simulink model "ScanMatcher_v21"  (R2021a)
settings: Solver=FixedStepAuto  StartTime=0.0  StopTime=inf  RelTol=1e-3
model workspace (MAT data in the model file):
  SL_ROS_VariableLengthArrays_MaxSizes : object (value not decoded)
undefined symbols (not defined in the file): Header, Pose, Theta, X, Y
libraries: robotlib x23, robotcorelib x2
(part 2 of 2)

== matlab function ScanMatcher_v21/Precise Localization/Compute Transformation/TrdICP_PP_corr/MATLAB Function4 ==
  data: data_set input size=[2,2000]; model_set input size=[2,2000]; N_d input size=1 [..2000]; N_m input size=1 [..2000]; iterCount output; R output; B_init input; maxIter input; T output; dev_A output; sigmaMult input; alphaIn input; scanTime input; ScanTime output
function [iterCount,R,T,dev_A,ScanTime] = FindTransform(data_set,model_set,N_d,N_m,B_init,maxIter,sigmaMult,alphaIn,scanTime)
%%%%%%%%%%%%%%%%%%%%%%%%%%%%%%%%%%%%%%%%%%%%%%%%%%%%%%%%%%%%%%%%%%%%%%%%%%%
%%%%%%%%%%%%%%%% Rigid ICP, Correntropy, Point to Point %%%%%%%%%%%%%%%%%%%
%%%%%%%%%%%%%%%%%%%%%%%%%%%%%%%%%%%%%%%%%%%%%%%%%%%%%%%%%%%%%%%%%%%%%%%%%%%
% Author  : Abdurrahman YILMAZ
% Date    : 15.09.2021
% Version : v01
% Notes   : ICP based 2D pose estimator. It takes model and data 
% clouds in 2D, target pose and initial pose information, and estimates 
% current pose
%%%%%%%%%%%%%%%%%%%%%%%%%%%%%%%%%%%%%%%%%%%%%%%%%%%%%%%%%%%%%%%%%%%%%%%%%%
    
    if isempty(maxIter) || isnan(maxIter) || isinf(maxIter) || maxIter <= 0 || maxIter >= 500
        maxNumIter = int32(100); % default value
    else
        maxNumIter = maxIter; % taken as ros paramter
    end
    
    if isempty(sigmaMult) || isnan(sigmaMult) || isinf(sigmaMult) || sigmaMult <= 0 || sigmaMult >= 100
        sigmaMultiplier = double(1); % default value
    else
        sigmaMultiplier = sigmaMult; % taken as ros paramter
    end
    
    if isempty(alphaIn) || isnan(alphaIn) || isinf(alphaIn) || alphaIn <= 0 || alphaIn >= 1
        alpha = double(0.8); % default value
    else
        alpha = alphaIn; % taken as ros paramter
    end
    
    sigma = 1;
    sigma_km1 = 0.1;
    B_km1 = B_init;
    B_k = B_init;
    count_stop_iter = 0;
    iterCount = int16(0);
    
    model_in = model_set';
    data_in = data_set';
    
%     N_model = nnz(~isnan(model_in))/2;
%     N_data = nnz(~isnan(data_in))/2;
    
    N_model = N_m;
    N_data = N_d;
    model= model_in(1:N_model,:);
    M1 = model;
    M = [M1,ones(size(M1,1),1)];
    data = data_in(1:N_data,:);
    P1 = data;
    P = [P1,ones(size(P1,1),1)];
    g = zeros(1,size(P1,1));
    
    p_k = zeros(size(P1,1),1);
    Q = zeros(size(P1,1),2);
    X = zeros(size(P1,1),2);
        
%     p_k = zeros(N_data,1);
    mck = [];
    P_trim = [];
    
    for iter = 1:maxNumIter
        iterCount = iterCount + 1;
        Pbar = (B_km1*P')';
        [Idx,Dist] = knnsearch(M(:,1:2),Pbar(:,1:2),'k',1);
        corr_points = [double(Idx),Dist,Pbar,P];
        corr_points = sortrows(corr_points,2);
        
        filterOutDist = median(Dist) + (median(Dist)-min(Dist));
        
        indexId = size(corr_points,1);
        
        for j = size(corr_points,1):-1:1
            if corr_points(j,2) <= filterOutDist
                indexId = j;
                break;
            end
        end
        Idx_filtered = corr_points(1:indexId,1);
        
        mck = [zeros(size(Idx_filtered,1),2),ones(size(Idx_filtered,1),1)];
        mck(:,1:2) = M(Idx_filtered,1:2);
        Pbar_trim = corr_points(1:indexId,3:4);
        P_trim = corr_points(1:indexId,6:8);
        
        DiffModelData = zeros(length(Pbar_trim),1);
        for i=1:1:length(Pbar_trim)
            DiffModelData(i,1)=sqrt((Pbar_trim(i,1)-mck(i,1))^2+(Pbar_trim(i,2)-mck(i,2))^2);
        end
%         if  iter < 100
%             sigma = sigmaMultiplier*std(DiffModelData);
%         else
%             sigma = sigma_km1*alpha + sigmaMultiplier*(1 - alpha)*sqrt(3/kurtosis(DiffModelData)*std(DiffModelData)^2); % 3 is standard Gaussian curve kurtosis 
%         end
        
        if iter ==1
            sigma = sigmaMultiplier*median(DiffModelData)*alpha + (1 - alpha)*sqrt(3/kurtosis(DiffModelData)*std(DiffModelData)^2);
        else
            sigma = sigma_km1*alpha;
        end
        
        for j = 1:1:size(P_trim,1)
            p_k(j) = exp(-(norm(B_km1*P_trim(j,:)'-mck(j,:)')^2/(2*sigma^2)));
        end
        
        sum_p_k_x = zeros(1,2);
        sum_p_k = 0;
        sum_p_k_y = zeros(1,2);
        
        for t = 1:1:size(P_trim,1)
            sum_p_k_x = sum_p_k_x + p_k(t)*P_trim(t,1:2);
            sum_p_k = sum_p_k + p_k(t);
            sum_p_k_y = sum_p_k_y + p_k(t)*mck(t,1:2);
        end
        
        Q_rem = sum_p_k_x/sum_p_k;
        X_rem = sum_p_k_y/sum_p_k;
        
        for tt = 1:1:size(P_trim,1)
            Q(tt,:) = P_trim(tt,1:2) - Q_rem;
            X(tt,:) = mck(tt,1:2) - X_rem;
        end
        
        for i = 1:1:size(P_trim,1)
            g(i) = exp(-(norm(B_km1*[Q(i,:)';1]-[X(i,:)';1])^2/(2*sigma^2)));
        end
        
        D_g = diag(g);
        Ltr_R = -(X'*D_g*Q)/(sigma^2);
        [U,~,Vtr] = svd(Ltr_R);
        if det(X'*D_g*Q) > 0
            D_d_inv = -eye(2);
        else
            D_d_inv = [1,0;0,-1];
        end
        R_k = U*D_d_inv*Vtr;
%         R_k = U*Vtr;
        
        if det(R_k) < 0
            Vtr(:,end) = -Vtr(:,end); 
            R_k = U*D_d_inv*Vtr;
        end
        
        sumForTk = zeros(2,1);
        for p = 1:1:size(P_trim,1)
            sumForTk = sumForTk + (mck(p,1:2)'-R_k*P_trim(p,1:2)')*p_k(p);
        end
        
        t_k = sumForTk/sum_p_k;
        B_k = [R_k,t_k;0,0,1];
%         B_k = [R_k*B_km1(1:2,1:2),R_k*B_km1(1:2,3)+t_k;zeros(1,2),ones(1,1)];
                
        if abs(norm(B_km1(1:3,1:3))-norm(B_k(1:3,1:3))) < 0.00005
            count_stop_iter = count_stop_iter + 1;
            if count_stop_iter > 5
                break;
            end
        else
            count_stop_iter = 0;
        end
        
        B_km1 = B_k(1:3,1:3);
        sigma_km1 = sigma;
    end
        
    B_final = B_k(1:3,1:3);
    
    % Rigid transformation R matrix and T vector
    R = B_final(1:2,1:2);
    T = B_final(1:2,3);
    dev_A = 0;
    iterCount = int16(iterCount);
    ScanTime = scanTime;

== matlab function ScanMatcher_v21/Precise Localization/OdomArray/MATLAB Function3 ==
  data: ScanEstimTime input; OdomArray input; xyth_odom output
function xyth_odom  = OdomUpdater(ScanEstimTime,OdomArray)

    scanTime = ScanEstimTime(1,1);
    
    estimTime = ScanEstimTime(2,1);
    
    indexOdomLast = 1;
    indexOdomFirst = 1;
    th = 0;
    x = 0;
    y = 0;
    
    for i = 1:1:size(OdomArray,1)
        if estimTime >= OdomArray(i,1)
            indexOdomLast = i;
            break;
        end
    end
    
    for i = 1:1:size(OdomArray,1)
        if scanTime >= OdomArray(i,1)
             indexOdomFirst = i;
             break;
        end
    end
    
    if indexOdomLast < indexOdomFirst
        for j = 0:1:indexOdomFirst-indexOdomLast
            if j == 0
                delta_t = OdomArray(indexOdomFirst - 1,1) - scanTime;
            elseif j == indexOdomFirst-indexOdomLast
                delta_t = estimTime - OdomArray(indexOdomLast,1);    
            else
                delta_t = OdomArray(indexOdomFirst - j - 1,1) - OdomArray(indexOdomFirst - j,1);
            end
            v_x = OdomArray(indexOdomFirst - j,2);
            w_z = OdomArray(indexOdomFirst - j,3);
            delta_x = v_x*cos(th)*delta_t;
            delta_y = v_x*sin(th)*delta_t;
            delta_th = w_z*delta_t;
            x = x + delta_x;
            y = y + delta_y;
            th = th + delta_th;
        end
    elseif indexOdomLast == indexOdomFirst
        delta_t = estimTime - scanTime;
        v_x = OdomArray(indexOdomFirst,2);
        w_z = OdomArray(indexOdomFirst,3);
        delta_x = v_x*cos(th)*delta_t;
        delta_y = v_x*sin(th)*delta_t;
        delta_th = w_z*delta_t;
        x = x + delta_x;
        y = y + delta_y;
        th = th + delta_th;
    end
   
%     odomDiff = odomLast - odomInit;
%     x_up = x + odomDiff(1,1);
%     y_up = y + odomDiff(1,1);
%     th_up = wrapTo360(th + odomDiff(1,1));
    
    xyth_odom = [x,y,th];
    
end

== matlab function ScanMatcher_v21/Precise Localization/Publish pose_estim_now_odom_updated (x,y,theta)/MATLAB Function3 ==
  data: x input; y input; x_up output; th input; xyth_odom input; y_up output; th_up output; R_th_up output
function [x_up,y_up,th_up,R_th_up]  = OdomUpdater(x,y,th,xyth_odom)

    xy_up = [cosd(th) -sind(th);sind(th) cosd(th)]*xyth_odom(1,1:2)' + [x;y];
    th_up = wrapTo360(th + rad2deg(xyth_odom(1,3)));
    x_up = xy_up(1,1);
    y_up = xy_up(2,1);
    R_th_up = rotz(th_up);
    
end

== matlab function ScanMatcher_v21/Precise Localization/Extract Model and Data Sets/MATLAB Function1 ==
  data: Sec input; sec output size=1 [..2000]; nSec input
function sec = TimeCalc(Sec,nSec)

    sec = Sec + 10^(-9)*nSec;
end

== matlab function ScanMatcher_v21/Precise Localization/Publish pose_estim_now_with_stamp (x,y,theta,time,frameID,...)/MATLAB Function1 ==
  data: ScanTime input; scanTime output; Sec input; estimTime output size=1 [..2000]; nSec input
function [scanTime,estimTime] = ScanvsEstimTime(ScanTime,Sec,nSec)

    estimTime = Sec + 10^(-9)*nSec;
    scanTime = ScanTime;
end

== matlab function ScanMatcher_v21/Precise Localization/Publish pose_estim_now_with_stamp (x,y,theta,time,frameID,...)/MATLAB Function2 ==
  data: dev_A input; covarianceMatrix output
function covarianceMatrix  = CovarianceEstim(dev_A)
    var_A = dev_A^2;
    x_cov = var_A;
    y_cov = var_A;
    z_cov = 0;
    rotx_cov = 0;
    roty_cov = 0;
    rotz_cov = var_A;

    covarianceMatrix = double([x_cov,0,0,0,0,0 ...
        0,y_cov,0,0,0,0,...
        0,0,z_cov,0,0,0,...
        0,0,0,rotx_cov,0,0,...
        0,0,0,0,roty_cov,0,...
        0,0,0,0,0,rotz_cov]);
end

== matlab function ScanMatcher_v21/Precise Localization/Publish pose_estim_now_odom_updated_with_stamp (x,y,theta,time,frameID,...)/MATLAB Function4 ==
  data: Rin input; x output; y output; z output; w output
function [x,y,z,w]  = Quat(Rin)
    w = Rin(1,1);
    x = Rin(2,1);
    y = Rin(3,1);
    z = Rin(4,1);
end

== matlab function ScanMatcher_v21/Precise Localization/Publish pose_estim_now_odom_updated_with_stamp (x,y,theta,time,frameID,...)/MATLAB Function2 ==
  data: dev_A input; covarianceMatrix output
function covarianceMatrix  = CovarianceEstim(dev_A)
    var_A = dev_A^2;
    x_cov = var_A;
    y_cov = var_A;
    z_cov = 0;
    rotx_cov = 0;
    roty_cov = 0;
    rotz_cov = var_A;

    covarianceMatrix = double([x_cov,0,0,0,0,0 ...
        0,y_cov,0,0,0,0,...
        0,0,z_cov,0,0,0,...
        0,0,0,rotx_cov,0,0,...
        0,0,0,0,roty_cov,0,...
        0,0,0,0,0,rotz_cov]);
end

== matlab function ScanMatcher_v21/Precise Localization/OdomArray/MATLAB Function5 ==
  data: pos_x input; pos_y input; pos_th input; Sec input; nSec input; vel_x input; vel_w_z input; ArrayOdomLast input; ArrayOdomNow output
function ArrayOdomNow  = OdomDataList(pos_x,pos_y,pos_th,Sec,nSec,vel_x,vel_w_z,ArrayOdomLast)

    sec = Sec + 10^(-9)*nSec;
    v_x = vel_x;
    w_z = vel_w_z;
    
    ArrayOdomDummy = ArrayOdomLast;
    
    if sec ~= ArrayOdomLast(1,1)
        ArrayOdomDummy = [sec,v_x,w_z,pos_x,pos_y,pos_th;ArrayOdomDummy(1:end-1,:)];
    end
    
    ArrayOdomNow = ArrayOdomDummy;
    
end

== matlab function ScanMatcher_v21/MATLAB Function8 ==
  data: docking_enable_msg input; docking_state output
function docking_state = Docking_State(docking_enable_msg)
    
    if isempty(docking_enable_msg) || isnan(docking_enable_msg)
        docking_state = false(1);
    else
        if docking_enable_msg
            docking_state = true(1);
        else
            docking_state = false(1);
        end
    end
end

== matlab function ScanMatcher_v21/Precise Localization/Target Pose - Initial Transform/MATLAB Function1 ==
  data: pose_target input; B_init output [..2000]; pose_estim_pre input
function B_init = Initial_tf(pose_target,pose_estim_pre)

    th_B = wrapTo360(pose_estim_pre(3,1)-pose_target(3,1));
%     R_B = [cosd(th_B),-sind(th_B);sind(th_B),cosd(th_B)];
    R_trgt2ref_cf = [cosd(pose_target(3,1)),-sind(pose_target(3,1));sind(pose_target(3,1)),cosd(pose_target(3,1))];
    t_B = R_trgt2ref_cf'*(pose_estim_pre(1:2,1) - pose_target(1:2,1));
%     B_init = [R_B,t_B;0,0,1];
    B_init = rotz(th_B);
    B_init(1:2,3) = t_B;

end

== matlab function ScanMatcher_v21/Precise Localization/Extract Model and Data Sets/MATLAB Function ==
  data: NumberOfPointsInScan input size=1 [..2000]; rangeMax input; rangeMin input; Ranges_data input; Ranges_model input; RangesXY_data output double size=[2,2000]; angle_min input; angle_inc input; RangesXY_model output size=[2,2000]; N_data output size=1 [..2000]; N_model output size=1 [..2000]
function [RangesXY_data,RangesXY_model,N_data,N_model] = Model_Data_Extract(NumberOfPointsInScan,rangeMax,rangeMin,Ranges_data,Ranges_model,angle_min,angle_inc)
    
    N_model = 0;
    N_data = 0;

    if ~isnan(NumberOfPointsInScan)
        Ranges_data(Ranges_data < rangeMin | Ranges_data > rangeMax) = NaN;
        Ranges_model(Ranges_model < rangeMin | Ranges_model > rangeMax) = NaN;
        Ranges_Used_data = double(Ranges_data');            
        RangesXY_data = NaN(2,size(Ranges_Used_data,2));
        Ranges_Used_model = double(Ranges_model');          
        RangesXY_model = NaN(2,size(Ranges_Used_model,2));
%         coder.varsize('RangesXY',[2,2000],[1,1])        
    
        for i = 1:1:NumberOfPointsInScan
            if isinf(Ranges_Used_data(1,i))
               Ranges_Used_data(1,i) = NaN;  
            end
            RangesXY_data(:,i) = Ranges_Used_data(1,i)*[cos(angle_min + angle_inc*(i-1));...
                sin(angle_min + angle_inc*(i-1))];
        end
        
        RangesXY_data = sortrows(RangesXY_data')';
        for i = 1:1:NumberOfPointsInScan
            if isnan(RangesXY_data(1,i))
                N_data = i-1;
                break;
            end
        end
        
        for i = 1:1:NumberOfPointsInScan
            if isinf(Ranges_Used_model(1,i))
               Ranges_Used_model(1,i) = NaN;  
            end
            RangesXY_model(:,i) = Ranges_Used_model(1,i)*[cos(angle_min + angle_inc*(i-1));...
                sin(angle_min + angle_inc*(i-1))];
        end
        
        RangesXY_model = sortrows(RangesXY_model')';
        for i = 1:1:NumberOfPointsInScan
            if isnan(RangesXY_model(1,i))
                N_model = i-1;
                break;
            end
        end
        
    else
        RangesXY_data = [];
        RangesXY_model = [];
    end

== matlab function ScanMatcher_v21/Precise Localization/Target Pose - Initial Transform/MATLAB Function2 ==
  data: quat_In input; theta output size=1 [..2000]
function theta = Quat2Euler(quat_In)

    eul = quat2eul(quat_In');
    eul_deg = rad2deg(eul);
    theta = eul_deg(1,1);
end

== matlab function ScanMatcher_v21/Precise Localization/Pose Estimator ==
  data: R input; t input; scanTime input; dev_A input; pose_estim_x output; pose_estim_y output; pose_estim_theta output; pose_target input; R_theta output; frameID output; leng_frameID output; ScanTime output; Dev_A output; frameID_in input; leng_frameID_in input
function [pose_estim_x,pose_estim_y,pose_estim_theta,R_theta,frameID,leng_frameID,ScanTime,Dev_A]  = PoseEstimator(R,t,scanTime,dev_A,pose_target,frameID_in,leng_frameID_in)
        
    Rot_deg = rad2deg(atan2(R(2,1),R(1,1)));
    Tr_meter = t;
    pose_estim_now = [[cosd(pose_target(3,1)) -sind(pose_target(3,1));...
        sind(pose_target(3,1)) cosd(pose_target(3,1))]*Tr_meter + pose_target(1:2,:);...
        wrapTo360(pose_target(3,1)+Rot_deg)];
    pose_estim_x = pose_estim_now(1,1);
    pose_estim_y = pose_estim_now(2,1);
    pose_estim_theta = pose_estim_now(3,1);
    R_theta = rotz(pose_estim_theta);
    if leng_frameID_in > 0 && sum(frameID_in) > 0
        frameID_now = convertCharsToStrings(char(frameID_in(1:leng_frameID_in)));
        leng_frameID = uint32(leng_frameID_in);
    else
        frameID_now = "base_link";
        leng_frameID = uint32(strlength(frameID_now));
    end
    
    frameID = frameID_now;
        
    ScanTime = scanTime;
    Dev_A = dev_A;
end

== matlab function ScanMatcher_v21/Precise Localization/Publish pose_estim_now_with_stamp (x,y,theta,time,frameID,...)/MATLAB Function4 ==
  data: Rin input; x output; y output; z output; w output
function [x,y,z,w]  = Quat(Rin)
    w = Rin(1,1);
    x = Rin(2,1);
    y = Rin(3,1);
    z = Rin(4,1);
end

== matlab function ScanMatcher_v21/Precise Localization/Extract Model and Data Sets/MATLAB Function5 ==
  data: angle_min input; NumOfPointInScan output size=1 [..2000]; angle_max input; angle_inc input; ScanResDeg output
function [NumOfPointInScan,ScanResDeg]  = ScanInfo(angle_min,angle_max,angle_inc)
    NumOfPointInScan = double(round(abs(angle_max - angle_min)/angle_inc)+1);
    ScanResDeg = angle_inc*180/pi;
end
